simulink model "PPC_scheme_04072024_a"  (R2023b)
settings: Solver=FixedStepAuto  StartTime=0.0  StopTime=10.0  FixedStep=0.00025  RelTol=1e-3
libraries: slpidlib x1
settings Model: Creator=borgn  LastModifiedBy=borgn
settings SolverCC: ConcurrentTasks=on  PositivePriorityOrder=on
settings OptimizationCC: BlockReduction=off  OptimizeBlockIOStorage=off
settings DebuggingCC: TasksWithSamePriorityMsg=none
settings HardwareCC: ProdBitPerLong=64  ProdLongLongMode=on  ProdHWDeviceType=Intel->x86-64 (Linux 64)
settings RTWCC: Description=Simulink Real-Time  SystemTargetFile=slrealtime.tlc  TemplateMakefile=slrealtime_default_tmf  Toolchain=Simulink Real-Time Toolchain  BuildConfiguration=Faster Runs  CodeExecutionProfiling=on  TargetLang=C++

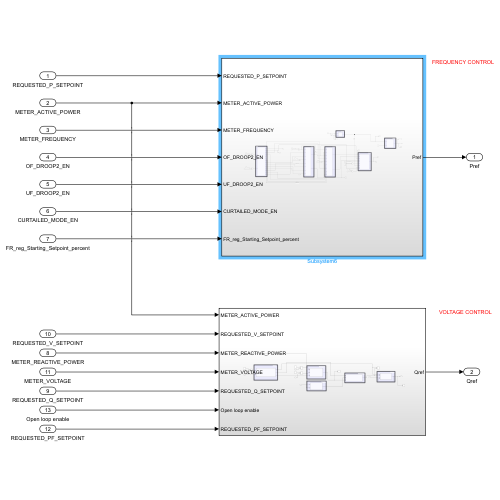
[thumbnail: Simulink's stored preview of the top-level diagram]
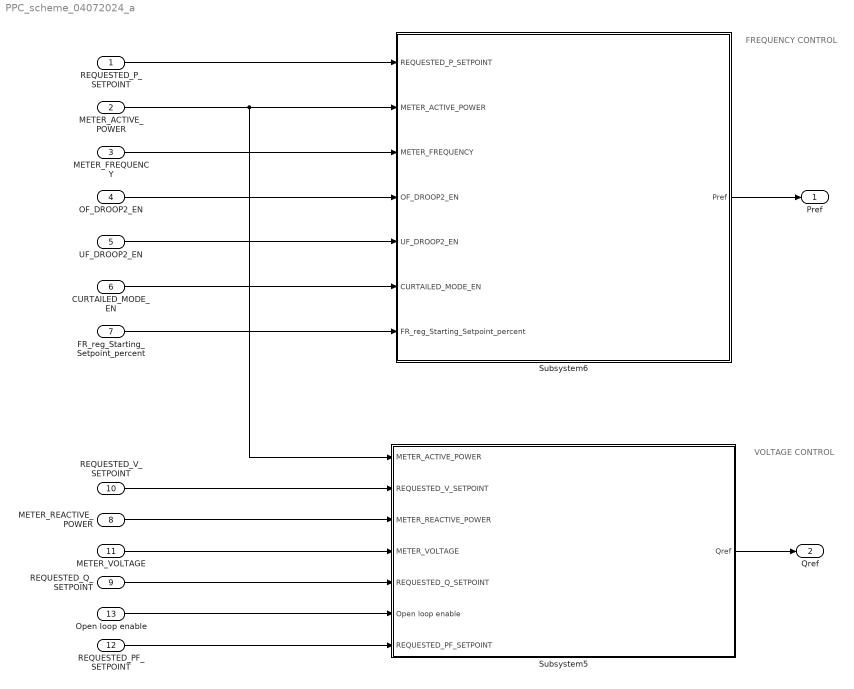
== system PPC_scheme_04072024_a ==
  note: FREQUENCY CONTROL
  note: VOLTAGE CONTROL
  REQUESTED_P_SETPOINT : Inport
  METER_ACTIVE_POWER : Inport  Port=2
  METER_FREQUENCY : Inport  Port=3
  OF_DROOP2_EN : Inport  Port=4
  UF_DROOP2_EN : Inport  Port=5
  CURTAILED_MODE_EN : Inport  Port=6
  FR_reg_Starting_Setpoint_percent : Inport  Port=7
  METER_REACTIVE_POWER : Inport  Port=8
  REQUESTED_Q_SETPOINT : Inport  Port=9
  REQUESTED_V_SETPOINT : Inport  Port=10
  METER_VOLTAGE : Inport  Port=11
  REQUESTED_PF_SETPOINT : Inport  Port=12
  Open loop enable : Inport  Port=13
  Subsystem5 : Subsystem
  Subsystem6 : Subsystem
  Pref : Outport
  Qref : Outport  Port=2
  wires:
  REQUESTED_P_SETPOINT/1 -> Subsystem6/1(REQUESTED_P_SETPOINT)
  METER_ACTIVE_POWER/1 -> Subsystem5/1(METER_ACTIVE_POWER), Subsystem6/2(METER_ACTIVE_POWER)
  METER_FREQUENCY/1 -> Subsystem6/3(METER_FREQUENCY)
  OF_DROOP2_EN/1 -> Subsystem6/4(OF_DROOP2_EN)
  UF_DROOP2_EN/1 -> Subsystem6/5(UF_DROOP2_EN)
  CURTAILED_MODE_EN/1 -> Subsystem6/6(CURTAILED_MODE_EN)
  FR_reg_Starting_Setpoint_percent/1 -> Subsystem6/7(FR_reg_Starting_Setpoint_percent)
  REQUESTED_V_SETPOINT/1 -> Subsystem5/2(REQUESTED_V_SETPOINT)
  METER_REACTIVE_POWER/1 -> Subsystem5/3(METER_REACTIVE_POWER)
  METER_VOLTAGE/1 -> Subsystem5/4(METER_VOLTAGE)
  REQUESTED_Q_SETPOINT/1 -> Subsystem5/5(REQUESTED_Q_SETPOINT)
  Open loop enable/1 -> Subsystem5/6(Open loop enable)
  REQUESTED_PF_SETPOINT/1 -> Subsystem5/7(REQUESTED_PF_SETPOINT)
  Subsystem6/1(Pref) -> Pref/1
  Subsystem5/1(Qref) -> Qref/1

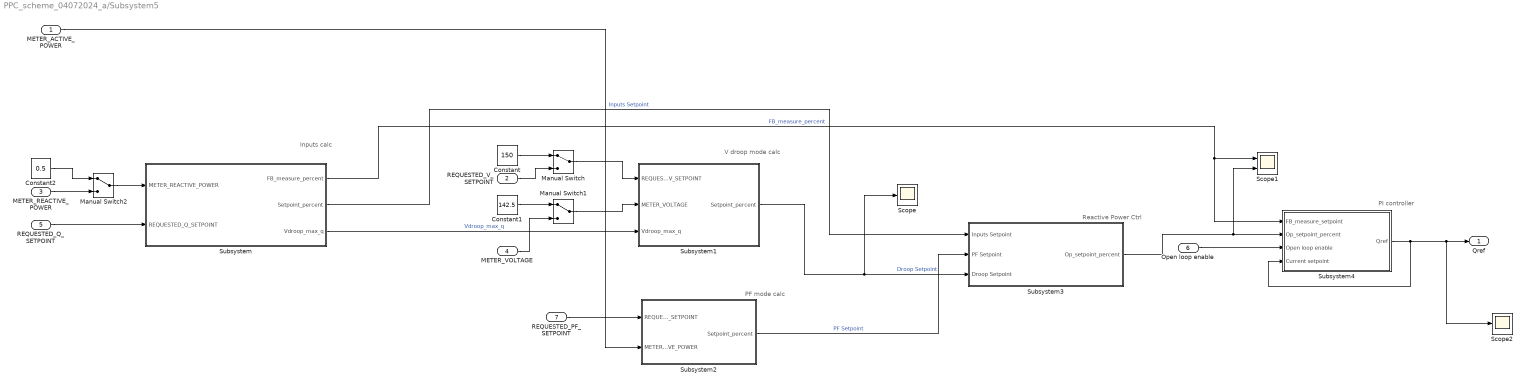
== system PPC_scheme_04072024_a/Subsystem5 ==
  note: PI controller
  note: Reactive Power Ctrl
  note: PF mode calc
  note: V droop mode calc
  note: Inputs calc
  METER_ACTIVE_POWER : Inport
  REQUESTED_V_SETPOINT : Inport  Port=2
  METER_REACTIVE_POWER : Inport  Port=3
  METER_VOLTAGE : Inport  Port=4
  REQUESTED_Q_SETPOINT : Inport  Port=5
  Open loop enable : Inport  Port=6
  REQUESTED_PF_SETPOINT : Inport  Port=7
  Constant : Constant  Value=150
  Constant1 : Constant  Value=142.5
  Constant2 : Constant  Value=0.5
  Manual Switch : ManualSwitch
  Manual Switch1 : ManualSwitch
  Manual Switch2 : ManualSwitch
  Scope : Scope
  Scope1 : Scope  NumInputPorts=2
  Scope2 : Scope
  Subsystem : Subsystem
  Subsystem1 : Subsystem
  Subsystem2 : Subsystem
  Subsystem3 : Subsystem
  Subsystem4 : Subsystem
  Qref : Outport
  wires:
  Subsystem/1(FB_measure_percent) -> Subsystem4/1(FB_measure_setpoint), Scope1/1  "FB_measure_percent"
  Subsystem4/1(Qref) -> Scope2/1, Qref/1, Subsystem4/4(Current setpoint)
  Subsystem/2(Setpoint_percent) -> Subsystem3/1(Inputs Setpoint)  "Inputs Setpoint"
  Subsystem1/1(Setpoint_percent) -> Scope/1, Subsystem3/3(Droop Setpoint)  "Droop Setpoint"
  REQUESTED_Q_SETPOINT/1 -> Subsystem/2(REQUESTED_Q_SETPOINT)
  Subsystem/3(Vdroop_max_q) -> Subsystem1/3(Vdroop_max_q)  "Vdroop_max_q"
  REQUESTED_PF_SETPOINT/1 -> Subsystem2/1(REQUESTED_PF_SETPOINT)
  Subsystem2/1(Setpoint_percent) -> Subsystem3/2(PF Setpoint)  "PF Setpoint"
  Subsystem3/1(Op_setpoint_percent) -> Scope1/2, Subsystem4/2(Op_setpoint_percent)
  Open loop enable/1 -> Subsystem4/3(Open loop enable)
  METER_ACTIVE_POWER/1 -> Subsystem2/2(METER_ACTIVE_POWER)
  REQUESTED_V_SETPOINT/1 -> Manual Switch/2
  Manual Switch/1 -> Subsystem1/1(REQUESTED_V_SETPOINT)
  Constant/1 -> Manual Switch/1
  Manual Switch1/1 -> Subsystem1/2(METER_VOLTAGE)
  METER_VOLTAGE/1 -> Manual Switch1/2
  Constant1/1 -> Manual Switch1/1
  METER_REACTIVE_POWER/1 -> Manual Switch2/2
  Manual Switch2/1 -> Subsystem/1(METER_REACTIVE_POWER)
  Constant2/1 -> Manual Switch2/1

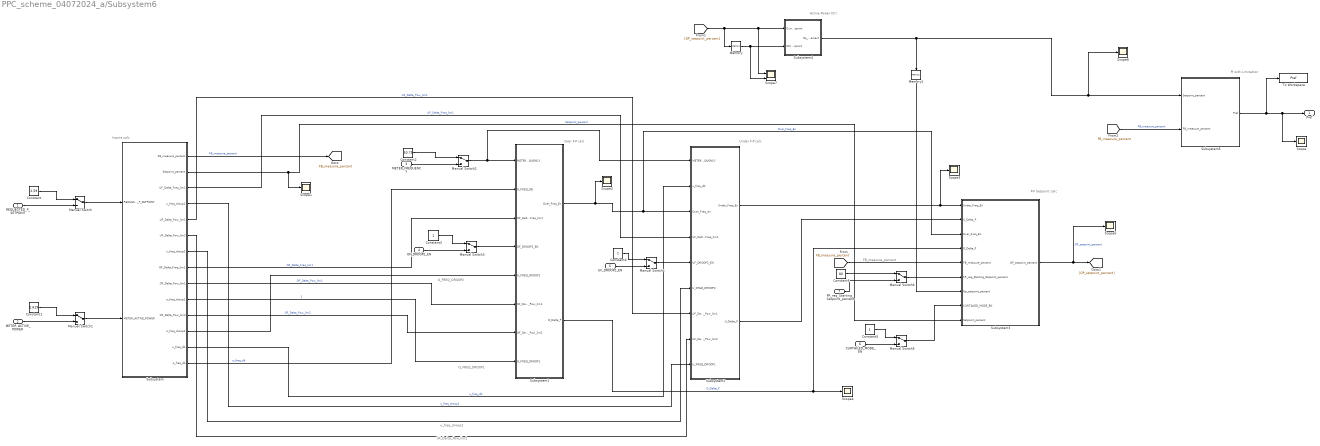
== system PPC_scheme_04072024_a/Subsystem6 ==
  note: PI with Limitation
  note: Active Power Ctrl
  note: FB_measure_percent
  note: P-F Setpoint calc
  note: UF_Delta_Pow_lim2
  note: u_freq_droop2
  note: Under F-P calc
  note: Inputs calc
  note: Over F-P calc
  note: O_FREQ_DROOP2
  note: O_FREQ_DROOP1
  REQUESTED_P_SETPOINT : Inport
  METER_ACTIVE_POWER : Inport  Port=2
  METER_FREQUENCY : Inport  Port=3
  OF_DROOP2_EN : Inport  Port=4
  UF_DROOP2_EN : Inport  Port=5
  CURTAILED_MODE_EN : Inport  Port=6
  FR_reg_Starting_Setpoint_percent : Inport  Port=7
  Constant : Constant  Value=2.59
  Constant1 : Constant  Value=1.619
  Constant2 : Constant  Value=50.75
  Constant3 : Constant
  Constant4 : Constant
  Constant5 : Constant
  Constant6 : Constant  Value=80
  Manual Switch{,1..6} (7 alike) : ManualSwitch
  Memory : Memory
  Memory1 : Memory
  Scope{,1..6} (7 alike) : Scope
  Scope7 : Scope  NumInputPorts=2
  Subsystem : Subsystem
  Subsystem1 : Subsystem
  Subsystem2 : Subsystem
  Subsystem3 : Subsystem
  Subsystem4 : Subsystem
  Subsystem5 : Subsystem
  To Workspace : ToWorkspace  VariableName=Pref  SaveFormat=Timeseries  SampleTime=-1
  Pref : Outport
  tag scope: FB_measure_percent=global
  wires:
  Constant1/1 -> Manual Switch1/1
  Manual Switch5/1 -> Subsystem3/8(CURTAILED_MODE_EN)
  Manual Switch6/1 -> Subsystem3/6(FR_reg_Starting_Setpoint_percent)
  Subsystem/11(OF_Delta_Pow_lim2) -> Subsystem1/7(OF_Delta_Pow_lim2)  "OF_Delta_Pow_lim2"
  CURTAILED_MODE_EN/1 -> Manual Switch5/2
  Manual Switch/1 -> Subsystem/1(REQUESTED_P_SETPOINT)
  Subsystem/9(OF_Delta_Pow_lim1) -> Subsystem1/6(OF_Delta_Pow_lim1)  "OF_Delta_Pow_lim1"
  Subsystem4/1(Op_setpoint_percent) -> Memory1/1, Scope6/1, Subsystem5/1(Setpoint_percent)
  Subsystem/1(FB_measure_percent) -> [FB_measure_percent]  "FB_measure_percent"
  Subsystem/14(o_freq_db) -> Subsystem1/2(O_FREQ_DB)  "o_freq_db"
  Subsystem/5(UF_Delta_Pow_lim1) -> Subsystem2/7(UF_Delta_Pow_lim1)  "UF_Delta_Pow_lim1"
  Subsystem2/1(Under_Freq_En) -> Scope3/1, Subsystem3/1(Under_Freq_En)
  Manual Switch1/1 -> Subsystem/2(METER_ACTIVE_POWER)
  [OP_setpoint_percent] -> Memory/1, Scope7/1, Subsystem4/1(Current Setpoint)
  OF_DROOP2_EN/1 -> Manual Switch3/2
  Subsystem/13(u_freq_db) -> Subsystem2/2(u_freq_db)  "u_freq_db"
  Memory1/1 -> Subsystem3/7(Op_setpoint_percent)
  Subsystem/12(o_freq_droop2) -> Subsystem1/5(O_FREQ_DROOP2)
  Subsystem/8(OF_Delta_Freq_lim1) -> Subsystem1/3(OF_Delta_Freq_lim1)  "OF_Delta_Freq_lim1"
  Constant5/1 -> Manual Switch5/1
  Subsystem5/1(Pref) -> To Workspace/1, Pref/1, Scope/1
  Constant/1 -> Manual Switch/1
  Manual Switch2/1 -> Subsystem2/1(METER_FREQUENCY), Subsystem1/1(METER_FREQUENCY)
  FR_reg_Starting_Setpoint_percent/1 -> Manual Switch6/2
  Subsystem/4(u_freq_droop1) -> Subsystem2/9(U_FREQ_DROOP1)  "u_freq_droop1"
  METER_ACTIVE_POWER/1 -> Manual Switch1/2
  UF_DROOP2_EN/1 -> Manual Switch4/2
  Subsystem/3(UF_Delta_Freq_lim1) -> Subsystem2/4(UF_Delta_Freq_lim1)  "UF_Delta_Freq_lim1"
  Subsystem/10(o_freq_droop1) -> Subsystem1/8(O_FREQ_DROOP1)  "1"
  REQUESTED_P_SETPOINT/1 -> Manual Switch/2
  Subsystem1/1(Over_Freq_En) -> Scope2/1, Subsystem3/3(Over_Freq_En), Subsystem2/3(Over_Freq_en)  "Over_Freq_En"
  [FB_measure_percent] -> Subsystem3/5(FB_measure_percent)
  [FB_measure_percent] -> Subsystem5/2(FB_measure_percent)  "FB_measure_percent"
  Manual Switch4/1 -> Subsystem2/5(UF_DROOP2_EN)
  METER_FREQUENCY/1 -> Manual Switch2/2
  Subsystem1/2(O_Delta_P) -> Subsystem3/4(O_Delta_P), Scope4/1  "O_Delta_P"
  Constant3/1 -> Manual Switch3/1
  Subsystem2/2(U_Delta_P) -> Subsystem3/2(U_Delta_P)
  Memory/1 -> Scope7/2, Subsystem4/2(Old Setpoint)
  Subsystem/6(UF_Delta_Pow_lim2) -> Subsystem2/8(UF_Delta_Pow_lim2)
  Constant2/1 -> Manual Switch2/1
  Constant4/1 -> Manual Switch4/1
  Subsystem/2(Setpoint_percent) -> Scope1/1, Subsystem3/9(Setpoint_percent)  "Setpoint_percent"
  Subsystem/7(u_freq_droop2) -> Subsystem2/6(U_FREQ_DROOP2)
  Manual Switch3/1 -> Subsystem1/4(OF_DROOP2_EN)
  Subsystem3/1(OP_setpoint_percent) -> Scope5/1, [OP_setpoint_percent]  "OP_setpoint_percent"
  Constant6/1 -> Manual Switch6/1

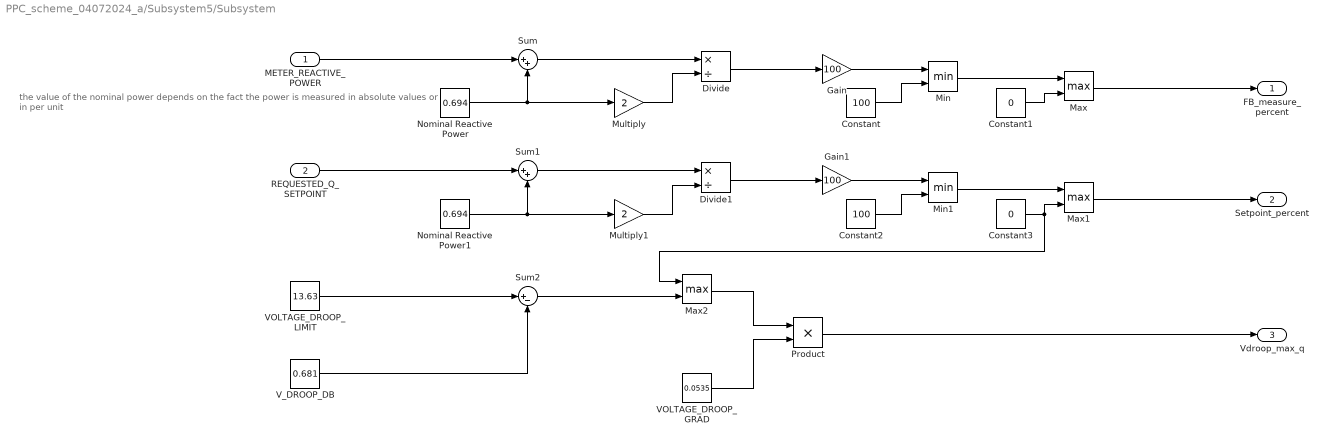
== system PPC_scheme_04072024_a/Subsystem5/Subsystem ==
  note: the value of the nominal power depends on the fact the power is measured in absolute values or in per unit
  METER_REACTIVE_POWER : Inport
  REQUESTED_Q_SETPOINT : Inport  Port=2
  Constant : Constant  Value=100
  Constant1 : Constant  Value=0
  Constant2 : Constant  Value=100
  Constant3 : Constant  Value=0
  Divide : Product  Inputs=*/
  Divide1 : Product  Inputs=*/
  Gain : Gain  Gain=100
  Gain1 : Gain  Gain=100
  Max : MinMax  Function=max  Inputs=2
  Max1 : MinMax  Function=max  Inputs=2
  Max2 : MinMax  Function=max  Inputs=2
  Min : MinMax  Inputs=2
  Min1 : MinMax  Inputs=2
  Multiply : Gain  Gain=2
  Multiply1 : Gain  Gain=2
  Nominal Reactive Power : Constant  Value=0.694
  Nominal Reactive Power1 : Constant  Value=0.694
  Product : Product
  Sum : Sum  Inputs=|++
  Sum1 : Sum  Inputs=|++
  Sum2 : Sum  Inputs=|+-
  VOLTAGE_DROOP_GRAD : Constant  Value=0.0535
  VOLTAGE_DROOP_LIMIT : Constant  Value=13.63
  V_DROOP_DB : Constant  Value=0.681
  FB_measure_percent : Outport
  Setpoint_percent : Outport  Port=2
  Vdroop_max_q : Outport  Port=3
  wires:
  Gain/1 -> Min/1
  Constant1/1 -> Max/2
  Max/1 -> FB_measure_percent/1
  Nominal Reactive Power/1 -> Multiply/1, Sum/2
  METER_REACTIVE_POWER/1 -> Sum/1
  Multiply/1 -> Divide/2
  Min/1 -> Max/1
  Sum/1 -> Divide/1
  Constant/1 -> Min/2
  Divide/1 -> Gain/1
  Multiply1/1 -> Divide1/2
  Constant2/1 -> Min1/2
  Sum1/1 -> Divide1/1
  REQUESTED_Q_SETPOINT/1 -> Sum1/1
  Nominal Reactive Power1/1 -> Multiply1/1, Sum1/2
  Min1/1 -> Max1/1
  Constant3/1 -> Max2/1, Max1/2
  Divide1/1 -> Gain1/1
  Gain1/1 -> Min1/1
  Max1/1 -> Setpoint_percent/1
  VOLTAGE_DROOP_LIMIT/1 -> Sum2/1
  V_DROOP_DB/1 -> Sum2/2
  Sum2/1 -> Max2/2
  Max2/1 -> Product/1
  VOLTAGE_DROOP_GRAD/1 -> Product/2
  Product/1 -> Vdroop_max_q/1

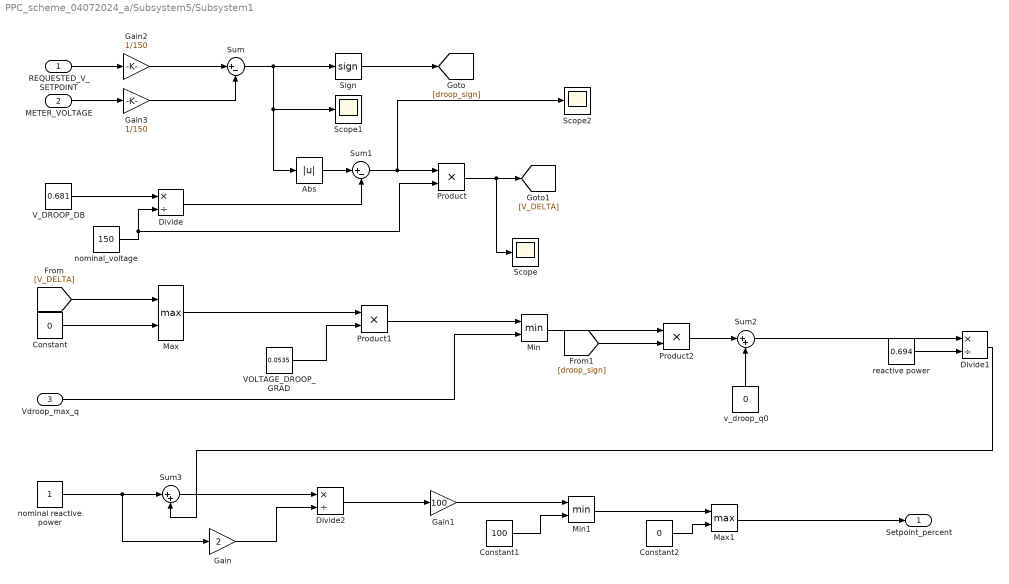
== system PPC_scheme_04072024_a/Subsystem5/Subsystem1 ==
  REQUESTED_V_SETPOINT : Inport
  METER_VOLTAGE : Inport  Port=2
  Vdroop_max_q : Inport  Port=3
  " reactive power" : Constant  Value=0.694
  Abs : Abs  SaturateOnIntegerOverflow=off
  Constant : Constant  Value=0
  Constant1 : Constant  Value=100
  Constant2 : Constant  Value=0
  Divide : Product  Inputs=*/
  Divide1 : Product  Inputs=*/
  Divide2 : Product  Inputs=*/
  Gain : Gain  Gain=2
  Gain1 : Gain  Gain=100
  Gain2 : Gain  Gain=1/150
  Gain3 : Gain  Gain=1/150
  Max : MinMax  Function=max  Inputs=2
  Max1 : MinMax  Function=max  Inputs=2
  Min : MinMax  Inputs=2
  Min1 : MinMax  Inputs=2
  Product : Product
  Product1 : Product
  Product2 : Product
  Scope : Scope
  Scope1 : Scope
  Scope2 : Scope
  Sign : Signum
  Sum : Sum  Inputs=|+-
  Sum1 : Sum  Inputs=|+-
  Sum2 : Sum  Inputs=|++
  Sum3 : Sum  Inputs=|++
  VOLTAGE_DROOP_GRAD : Constant  Value=0.0535
  V_DROOP_DB : Constant  Value=0.681
  nominal reactive power : Constant
  nominal_voltage : Constant  Value=150
  v_droop_q0 : Constant  Value=0
  Setpoint_percent : Outport
  wires:
  V_DROOP_DB/1 -> Divide/1
  Constant/1 -> Max/2
  Divide/1 -> Sum1/2
  Sum1/1 -> Scope2/1, Product/1
  nominal_voltage/1 -> Product/2, Divide/2
  Abs/1 -> Sum1/1
  Product/1 -> Scope/1, [V_DELTA]
  [V_DELTA] -> Max/1
  Sign/1 -> [droop_sign]
  Max/1 -> Product1/1
  VOLTAGE_DROOP_GRAD/1 -> Product1/2
  Product1/1 -> Min/1
  Vdroop_max_q/1 -> Min/2
  Min/1 -> Product2/1
  [droop_sign] -> Product2/2
  Product2/1 -> Sum2/1
  v_droop_q0/1 -> Sum2/2
  Sum2/1 -> Divide1/1
  " reactive power"/1 -> Divide1/2
  Divide1/1 -> Sum3/2
  nominal reactive power/1 -> Gain/1, Sum3/1
  Sum3/1 -> Divide2/1
  Gain/1 -> Divide2/2
  Divide2/1 -> Gain1/1
  Gain1/1 -> Min1/1
  Constant1/1 -> Min1/2
  Min1/1 -> Max1/1
  Constant2/1 -> Max1/2
  Max1/1 -> Setpoint_percent/1
  REQUESTED_V_SETPOINT/1 -> Gain2/1
  METER_VOLTAGE/1 -> Gain3/1
  Gain2/1 -> Sum/1
  Gain3/1 -> Sum/2
  Sum/1 -> Abs/1, Scope1/1, Sign/1

== system PPC_scheme_04072024_a/Subsystem5/Subsystem2 ==
  REQUESTED_PF_SETPOINT : Inport
  METER_ACTIVE_POWER : Inport  Port=2
  Constant : Constant  Value=100
  Constant1 : Constant  Value=0
  Divide : Product  Inputs=*/
  Divide1 : Product  Inputs=*/
  Gain : Gain  Gain=2
  Gain1 : Gain  Gain=100
  Max : MinMax  Function=max  Inputs=2
  Min : MinMax  Inputs=2
  Product : Product
  Sin : Trigonometry  Operator=acos
  Sum : Sum  Inputs=|++
  Tan : Trigonometry  Operator=tan
  nominal active power : Constant  Value=3.238
  nominal reactive power : Constant
  Setpoint_percent : Outport
  wires:
  REQUESTED_PF_SETPOINT/1 -> Sin/1
  METER_ACTIVE_POWER/1 -> Divide/1
  Sin/1 -> Tan/1
  nominal active power/1 -> Divide/2
  Tan/1 -> Product/1
  Divide/1 -> Product/2
  Product/1 -> Sum/1
  nominal reactive power/1 -> Gain/1, Sum/2
  Sum/1 -> Divide1/1
  Gain/1 -> Divide1/2
  Divide1/1 -> Gain1/1
  Gain1/1 -> Min/2
  Constant/1 -> Min/1
  Min/1 -> Max/1
  Constant1/1 -> Max/2
  Max/1 -> Setpoint_percent/1

== system PPC_scheme_04072024_a/Subsystem5/Subsystem3 ==
  Inputs Setpoint : Inport
  PF Setpoint : Inport  Port=2
  Droop Setpoint : Inport  Port=3
  MATLAB Function : MATLAB Function  TreatAsAtomicUnit=on
  Mux : Mux
  control mode : Constant  Value=3
  Op_setpoint_percent : Outport
  wires:
  MATLAB Function/1(y) -> Op_setpoint_percent/1
  Inputs Setpoint/1 -> Mux/2
  Mux/1 -> MATLAB Function/1(u)
  PF Setpoint/1 -> Mux/3
  Droop Setpoint/1 -> Mux/4
  control mode/1 -> Mux/1

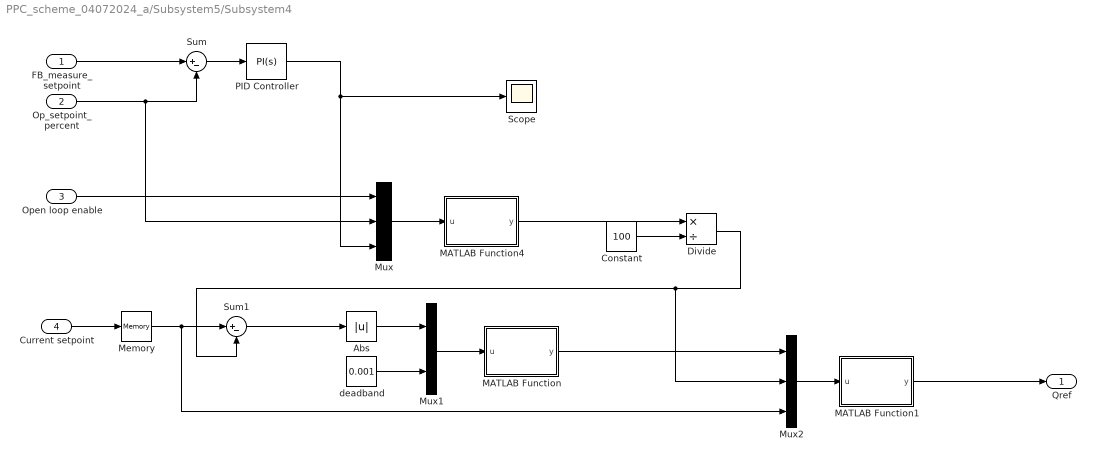
== system PPC_scheme_04072024_a/Subsystem5/Subsystem4 ==
  FB_measure_setpoint : Inport
  Op_setpoint_percent : Inport  Port=2
  Open loop enable : Inport  Port=3
  Current setpoint : Inport  Port=4
  Abs : Abs  SaturateOnIntegerOverflow=off
  Constant : Constant  Value=100
  Divide : Product  Inputs=*/
  MATLAB Function : MATLAB Function  TreatAsAtomicUnit=on
  MATLAB Function1 : MATLAB Function  TreatAsAtomicUnit=on
  MATLAB Function4 : MATLAB Function  TreatAsAtomicUnit=on
  Memory : Memory
  Mux : Mux  Inputs=3
  Mux1 : Mux  Inputs=2
  Mux2 : Mux  Inputs=3
  PID Controller : slpidlib/PID Controller  Controller=PI  Form=Parallel  TimeDomain=Continuous-time  UseExternalTs=off  SampleTime=-1  IntegratorMethod=Forward Euler  FilterMethod=Forward Euler  ControllerParametersSource=internal  P=1  I=0.05  UseKiTs=off  D=0  N=100  UseFilter=on  TunerSelectOption=Transfer Function Based (PID Tuner App)  InitialConditionSource=internal  InitialConditionForIntegrator=0  InitialConditionForFilter=0  DifferentiatorICPrevScaledInput=0  ExternalReset=none  TrackingMode=off  Kt=1  LimitOutput=on  SatLimitsSource=internal  UpperSaturationLimit=100  LowerSaturationLimit=-100  LinearizeAsGain=on  AntiWindupMode=none  Kb=1  LimitIntegrator=off  UpperIntegratorSaturationLimit=inf  LowerIntegratorSaturationLimit=-inf  POutMin=[]  POutMax=[]  IOutMin=[]  IOutMax=[]  DOutMin=[]  DOutMax=[]  NOutMin=[]  NOutMax=[]  SumOutMin=[]  SumOutMax=[]  SaturationOutMin=[]  SaturationOutMax=[]  PParamMin=[]  PParamMax=[]  IParamMin=[]  IParamMax=[]  DParamMin=[]  DParamMax=[]  NParamMin=[]  NParamMax=[]  KbParamMin=[]  KbParamMax=[]  KtParamMin=[]  KtParamMax=[]  KbOutMin=[]  KbOutMax=[]  KtOutMin=[]  KtOutMax=[]  IntegratorOutMin=[]  IntegratorOutMax=[]  FilterOutMin=[]  FilterOutMax=[]  SumI1OutMin=[]  SumI1OutMax=[]  SumI2OutMin=[]  SumI2OutMax=[]  SumI3OutMin=[]  SumI3OutMax=[]  SumI4OutMin=[]  SumI4OutMax=[]  SumDOutMin=[]  SumDOutMax=[]  DifferentiatorOutMin=[]  DifferentiatorOutMax=[]  FilterDiffOutCoefMin=[]  FilterDiffOutCoefMax=[]  ReciprocalOutMin=[]  ReciprocalOutMax=[]  SumDenOutMin=[]  SumDenOutMax=[]  SumNumOutMin=[]  SumNumOutMax=[]  DivideOutMin=[]  DivideOutMax=[]  UdiffTsProdOutMin=[]  UdiffTsProdOutMax=[]  NTsProdOutMin=[]  NTsProdOutMax=[]  UintegralTsProdOutMin=[]  UintegralTsProdOutMax=[]  UngainTsProdOutMin=[]  UngainTsProdOutMax=[]  ClampingZeroOutDataTypeStr=Inherit: Inherit via back propagation  ClampingZeroOutMin=[]  ClampingZeroOutMax=[]  FilterDenConstantOutDataTypeStr=Inherit: Inherit via back propagation  FilterDenConstantOutMin=[]  FilterDenConstantOutMax=[]  PCopyOutDataTypeStr=Inherit: Inherit via back propagation  PCopyOutMin=[]  PCopyOutMax=[]  NCopyOutDataTypeStr=Inherit: Inherit via back propagation  NCopyOutMin=[]  NCopyOutMax=[]  IntegratorContinuousStateAttributes=''  IntegratorStateMustResolveToSignalObject=off  IntegratorRTWStateStorageClass=Auto  FilterContinuousStateAttributes=''  FilterStateMustResolveToSignalObject=off  FilterRTWStateStorageClass=Auto  ParallelPVariant=InternalParameters  IdealPVariant=Disabled  IVariant=InternalParameters  DVariant=Disabled  IntegratorVariant=Continuous  SatVariant=Enabled  AWVariant=Passthrough  PCopyVariant=Disabled  TRVariant=Disabled  FdbkBlocksVariant=Forward  IdealPFdbkVariant=Disabled  SatFdbkVariant=Disabled  DerivativeFilterVariant=Disabled  NVariant=Disabled  NCopyVariant=Disabled_SignalSpec  FilterICVariant=Disabled  IntegratorICVariant=InternalICs  ExternalResetVariant=Disabled  TRSumVariant=Passthrough  SumFdbkVariant=Disabled  SumVariant=Sum_PI  TsampFilterVariant=InternalTs  TsampNgainVariant=Passthrough  TsampIntegralVariant=Disabled_SignalSpec  ExternalSaturationOutDataTypeStr=Inherit: Same as second input
  Scope : Scope
  Sum : Sum  Inputs=|+-
  Sum1 : Sum  Inputs=|+-
  deadband : Constant  Value=0.001
  Qref : Outport
  wires:
  Op_setpoint_percent/1 -> Mux/2, Sum/2
  Sum/1 -> PID Controller/1
  FB_measure_setpoint/1 -> Sum/1
  PID Controller/1 -> Scope/1, Mux/3
  Open loop enable/1 -> Mux/1
  Mux/1 -> MATLAB Function4/1(u)
  MATLAB Function4/1(y) -> Divide/1
  Constant/1 -> Divide/2
  Divide/1 -> Mux2/2, Sum1/2
  Sum1/1 -> Abs/1
  Abs/1 -> Mux1/1
  deadband/1 -> Mux1/2
  Mux1/1 -> MATLAB Function/1(u)
  MATLAB Function/1(y) -> Mux2/1
  Mux2/1 -> MATLAB Function1/1(u)
  MATLAB Function1/1(y) -> Qref/1
  Current setpoint/1 -> Memory/1
  Memory/1 -> Mux2/3, Sum1/1

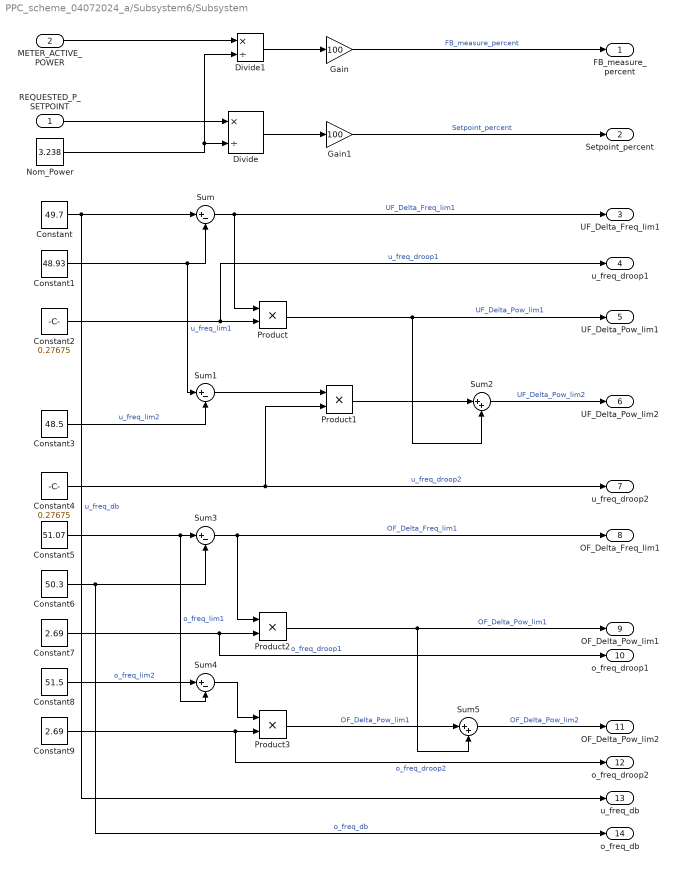
== system PPC_scheme_04072024_a/Subsystem6/Subsystem ==
  REQUESTED_P_SETPOINT : Inport
  METER_ACTIVE_POWER : Inport  Port=2
  Constant : Constant  Value=49.7
  Constant1 : Constant  Value=48.93
  Constant2 : Constant  Value=0.27675
  Constant3 : Constant  Value=48.5
  Constant4 : Constant  Value=0.27675
  Constant5 : Constant  Value=51.07
  Constant6 : Constant  Value=50.3
  Constant7 : Constant  Value=2.69
  Constant8 : Constant  Value=51.5
  Constant9 : Constant  Value=2.69
  Divide : Product  Inputs=*/
  Divide1 : Product  Inputs=*/
  Gain : Gain  Gain=100
  Gain1 : Gain  Gain=100
  Nom_Power : Constant  Value=3.238
  Product{,1..3} (4 alike) : Product
  Sum{,1,3..4} (4 alike) : Sum  Inputs=|+-
  Sum2 : Sum  Inputs=|++
  Sum5 : Sum  Inputs=|++
  FB_measure_percent : Outport
  Setpoint_percent : Outport  Port=2
  UF_Delta_Freq_lim1 : Outport  Port=3
  u_freq_droop1 : Outport  Port=4
  UF_Delta_Pow_lim1 : Outport  Port=5
  UF_Delta_Pow_lim2 : Outport  Port=6
  u_freq_droop2 : Outport  Port=7
  OF_Delta_Freq_lim1 : Outport  Port=8
  OF_Delta_Pow_lim1 : Outport  Port=9
  o_freq_droop1 : Outport  Port=10
  OF_Delta_Pow_lim2 : Outport  Port=11
  o_freq_droop2 : Outport  Port=12
  u_freq_db : Outport  Port=13
  o_freq_db : Outport  Port=14
  wires:
  Gain/1 -> FB_measure_percent/1  "FB_measure_percent"
  Constant5/1 -> Sum4/2, Sum3/1  "o_freq_lim1"
  Sum/1 -> UF_Delta_Freq_lim1/1, Product/1  "UF_Delta_Freq_lim1"
  REQUESTED_P_SETPOINT/1 -> Divide/1
  Constant7/1 -> o_freq_droop1/1, Product2/2  "o_freq_droop1"
  Product/1 -> UF_Delta_Pow_lim1/1, Sum2/2  "UF_Delta_Pow_lim1"
  Sum5/1 -> OF_Delta_Pow_lim2/1  "OF_Delta_Pow_lim2"
  Nom_Power/1 -> Divide1/2, Divide/2
  Product2/1 -> OF_Delta_Pow_lim1/1, Sum5/2  "OF_Delta_Pow_lim1"
  Constant9/1 -> o_freq_droop2/1, Product3/2  "o_freq_droop2"
  Product1/1 -> Sum2/1
  Sum2/1 -> UF_Delta_Pow_lim2/1  "UF_Delta_Pow_lim2"
  Constant4/1 -> u_freq_droop2/1, Product1/2  "u_freq_droop2"
  Sum4/1 -> Product3/1
  Constant2/1 -> u_freq_droop1/1, Product/2  "u_freq_droop1"
  Constant1/1 -> Sum1/1, Sum/2  "u_freq_lim1"
  Product3/1 -> Sum5/1  "OF_Delta_Pow_lim1"
  Constant6/1 -> o_freq_db/1, Sum3/2  "o_freq_db"
  METER_ACTIVE_POWER/1 -> Divide1/1
  Constant/1 -> u_freq_db/1, Sum/1  "u_freq_db"
  Gain1/1 -> Setpoint_percent/1  "Setpoint_percent"
  Divide/1 -> Gain1/1
  Divide1/1 -> Gain/1
  Sum1/1 -> Product1/1
  Constant3/1 -> Sum1/2  "u_freq_lim2"
  Sum3/1 -> OF_Delta_Freq_lim1/1, Product2/1  "OF_Delta_Freq_lim1"
  Constant8/1 -> Sum4/1  "o_freq_lim2"

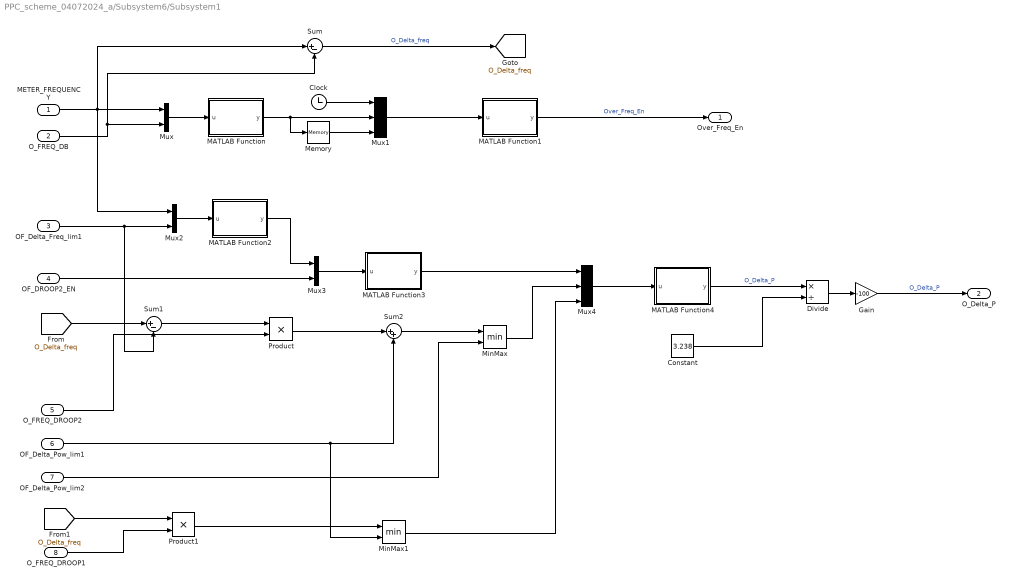
== system PPC_scheme_04072024_a/Subsystem6/Subsystem1 ==
  METER_FREQUENCY : Inport
  O_FREQ_DB : Inport  Port=2
  OF_Delta_Freq_lim1 : Inport  Port=3
  OF_DROOP2_EN : Inport  Port=4
  O_FREQ_DROOP2 : Inport  Port=5
  OF_Delta_Pow_lim1 : Inport  Port=6
  OF_Delta_Pow_lim2 : Inport  Port=7
  O_FREQ_DROOP1 : Inport  Port=8
  Clock : Clock
  Constant : Constant  Value=3.238
  Divide : Product  Inputs=*/
  Gain : Gain  Gain=-100
  MATLAB Function : MATLAB Function  TreatAsAtomicUnit=on
  MATLAB Function1 : MATLAB Function  TreatAsAtomicUnit=on
  MATLAB Function2 : MATLAB Function  TreatAsAtomicUnit=on
  MATLAB Function3 : MATLAB Function  TreatAsAtomicUnit=on
  MATLAB Function4 : MATLAB Function  TreatAsAtomicUnit=on
  Memory : Memory
  MinMax : MinMax  Inputs=2
  MinMax1 : MinMax  Inputs=2
  Mux : Mux  Inputs=2
  Mux1 : Mux  Inputs=3
  Mux2 : Mux  Inputs=2
  Mux3 : Mux  Inputs=2
  Mux4 : Mux  Inputs=3
  Product : Product
  Product1 : Product
  Sum : Sum  Inputs=|+-
  Sum1 : Sum  Inputs=|+-
  Sum2 : Sum  Inputs=|++
  Over_Freq_En : Outport
  O_Delta_P : Outport  Port=2
  tag scope: O_Delta_freq=global
  wires:
  Memory/1 -> Mux1/3
  Sum1/1 -> Product/1
  OF_Delta_Pow_lim2/1 -> MinMax/2
  OF_Delta_Pow_lim1/1 -> MinMax1/2, Sum2/2
  Sum/1 -> [O_Delta_freq]  "O_Delta_freq"
  Mux1/1 -> MATLAB Function1/1(u)
  MATLAB Function/1(y) -> Memory/1, Mux1/2
  Mux3/1 -> MATLAB Function3/1(u)
  MATLAB Function3/1(y) -> Mux4/1
  OF_Delta_Freq_lim1/1 -> Sum1/2, Mux2/2
  Clock/1 -> Mux1/1
  METER_FREQUENCY/1 -> Mux2/1, Sum/1, Mux/1
  Mux/1 -> MATLAB Function/1(u)
  MinMax1/1 -> Mux4/3
  O_FREQ_DROOP2/1 -> Product/2
  OF_DROOP2_EN/1 -> Mux3/2
  MATLAB Function2/1(y) -> Mux3/1
  O_FREQ_DROOP1/1 -> Product1/2
  O_FREQ_DB/1 -> Sum/2, Mux/2
  MATLAB Function1/1(y) -> Over_Freq_En/1  "Over_Freq_En"
  Mux2/1 -> MATLAB Function2/1(u)
  Mux4/1 -> MATLAB Function4/1(u)
  [O_Delta_freq] -> Sum1/1
  Sum2/1 -> MinMax/1
  Product1/1 -> MinMax1/1
  MinMax/1 -> Mux4/2
  Product/1 -> Sum2/1
  [O_Delta_freq] -> Product1/1
  MATLAB Function4/1(y) -> Divide/1  "O_Delta_P"
  Constant/1 -> Divide/2
  Divide/1 -> Gain/1
  Gain/1 -> O_Delta_P/1  "O_Delta_P"

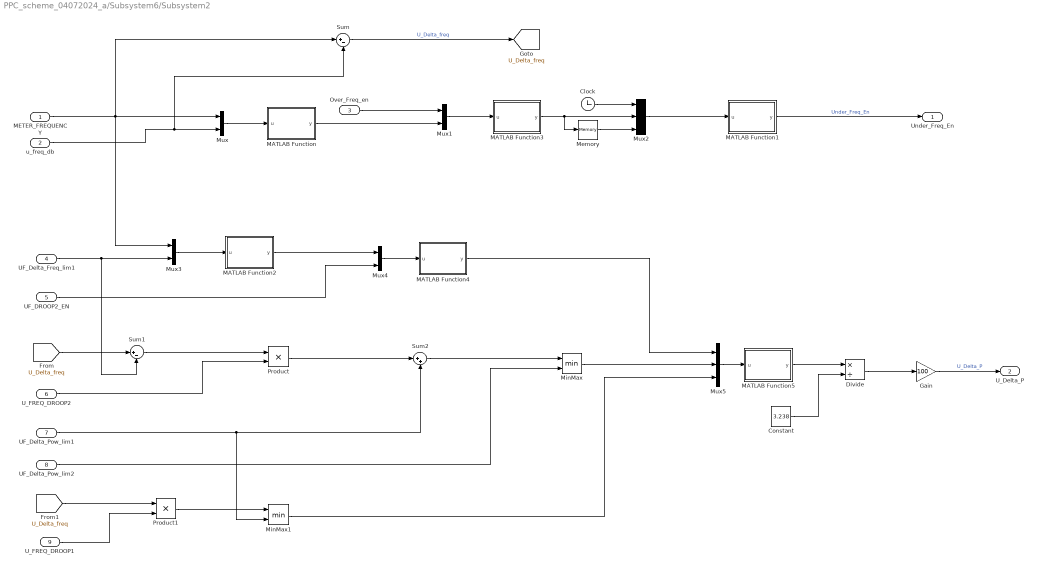
== system PPC_scheme_04072024_a/Subsystem6/Subsystem2 ==
  METER_FREQUENCY : Inport
  u_freq_db : Inport  Port=2
  Over_Freq_en : Inport  Port=3
  UF_Delta_Freq_lim1 : Inport  Port=4
  UF_DROOP2_EN : Inport  Port=5
  U_FREQ_DROOP2 : Inport  Port=6
  UF_Delta_Pow_lim1 : Inport  Port=7
  UF_Delta_Pow_lim2 : Inport  Port=8
  U_FREQ_DROOP1 : Inport  Port=9
  Clock : Clock
  Constant : Constant  Value=3.238
  Divide : Product  Inputs=*/
  Gain : Gain  Gain=100
  MATLAB Function : MATLAB Function  TreatAsAtomicUnit=on
  MATLAB Function1 : MATLAB Function  TreatAsAtomicUnit=on
  MATLAB Function2 : MATLAB Function  TreatAsAtomicUnit=on
  MATLAB Function3 : MATLAB Function  TreatAsAtomicUnit=on
  MATLAB Function4 : MATLAB Function  TreatAsAtomicUnit=on
  MATLAB Function5 : MATLAB Function  TreatAsAtomicUnit=on
  Memory : Memory
  MinMax : MinMax  Inputs=2
  MinMax1 : MinMax  Inputs=2
  Mux{,1,3..4} (4 alike) : Mux  Inputs=2
  Mux2 : Mux  Inputs=3
  Mux5 : Mux  Inputs=3
  Product : Product
  Product1 : Product
  Sum : Sum  Inputs=|+-
  Sum1 : Sum  Inputs=|+-
  Sum2 : Sum  Inputs=|++
  Under_Freq_En : Outport
  U_Delta_P : Outport  Port=2
  tag scope: U_Delta_freq=global
  wires:
  Mux/1 -> MATLAB Function/1(u)
  u_freq_db/1 -> Sum/2, Mux/2
  METER_FREQUENCY/1 -> Mux3/1, Sum/1, Mux/1
  MATLAB Function/1(y) -> Mux1/2
  Over_Freq_en/1 -> Mux1/1
  Mux1/1 -> MATLAB Function3/1(u)
  MATLAB Function1/1(y) -> Under_Freq_En/1  "Under_Freq_En"
  Clock/1 -> Mux2/1
  Memory/1 -> Mux2/3
  MATLAB Function3/1(y) -> Memory/1, Mux2/2
  Mux2/1 -> MATLAB Function1/1(u)
  Sum/1 -> [U_Delta_freq]  "U_Delta_freq"
  UF_Delta_Freq_lim1/1 -> Sum1/2, Mux3/2
  Mux3/1 -> MATLAB Function2/1(u)
  MATLAB Function2/1(y) -> Mux4/1
  UF_DROOP2_EN/1 -> Mux4/2
  Mux4/1 -> MATLAB Function4/1(u)
  [U_Delta_freq] -> Sum1/1
  Sum1/1 -> Product/1
  U_FREQ_DROOP2/1 -> Product/2
  Product/1 -> Sum2/1
  UF_Delta_Pow_lim1/1 -> MinMax1/2, Sum2/2
  Sum2/1 -> MinMax/1
  UF_Delta_Pow_lim2/1 -> MinMax/2
  [U_Delta_freq] -> Product1/1
  U_FREQ_DROOP1/1 -> Product1/2
  Product1/1 -> MinMax1/1
  MATLAB Function4/1(y) -> Mux5/1
  MinMax/1 -> Mux5/2
  MinMax1/1 -> Mux5/3
  Mux5/1 -> MATLAB Function5/1(u)
  MATLAB Function5/1(y) -> Divide/1
  Constant/1 -> Divide/2
  Divide/1 -> Gain/1
  Gain/1 -> U_Delta_P/1  "U_Delta_P"

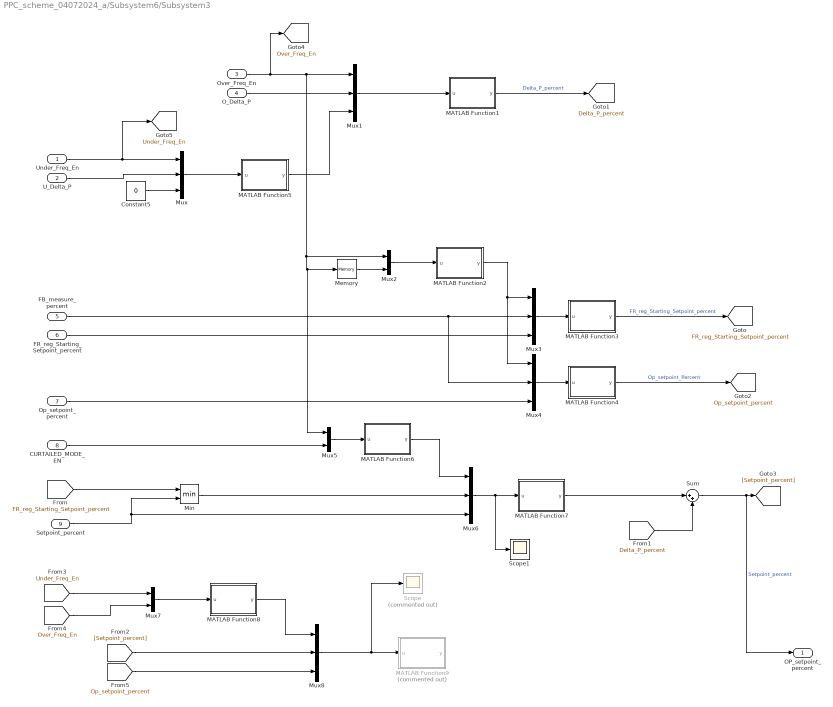
== system PPC_scheme_04072024_a/Subsystem6/Subsystem3 ==
  Under_Freq_En : Inport
  U_Delta_P : Inport  Port=2
  Over_Freq_En : Inport  Port=3
  O_Delta_P : Inport  Port=4
  FB_measure_percent : Inport  Port=5
  FR_reg_Starting_Setpoint_percent : Inport  Port=6
  Op_setpoint_percent : Inport  Port=7
  CURTAILED_MODE_EN : Inport  Port=8
  Setpoint_percent : Inport  Port=9
  Constant5 : Constant  Value=0
  MATLAB Function1 : MATLAB Function  TreatAsAtomicUnit=on
  MATLAB Function2 : MATLAB Function  TreatAsAtomicUnit=on
  MATLAB Function3 : MATLAB Function  TreatAsAtomicUnit=on
  MATLAB Function4 : MATLAB Function  TreatAsAtomicUnit=on
  MATLAB Function5 : MATLAB Function  TreatAsAtomicUnit=on
  MATLAB Function6 : MATLAB Function  TreatAsAtomicUnit=on
  MATLAB Function7 : MATLAB Function  TreatAsAtomicUnit=on
  MATLAB Function8 : MATLAB Function  TreatAsAtomicUnit=on
  MATLAB Function9 : MATLAB Function  Commented=on  TreatAsAtomicUnit=on
  Memory : Memory
  Min : MinMax  Inputs=2
  Mux{,1,3..4,6,8} (6 alike) : Mux  Inputs=3
  Mux2 : Mux  Inputs=2
  Mux5 : Mux  Inputs=2
  Mux7 : Mux  Inputs=2
  Scope : Scope  Commented=on
  Scope1 : Scope
  Sum : Sum  Inputs=|++
  OP_setpoint_percent : Outport
  tag scope: Delta_P_percent=global, FR_reg_Starting_Setpoint_percent=global, Op_setpoint_percent=global, Over_Freq_En=global, Under_Freq_En=global
  wires:
  Constant5/1 -> Mux/3
  Mux/1 -> MATLAB Function5/1(u)
  Under_Freq_En/1 -> [Under_Freq_En], Mux/1
  U_Delta_P/1 -> Mux/2
  Mux1/1 -> MATLAB Function1/1(u)
  Over_Freq_En/1 -> [Over_Freq_En], Mux1/1, Mux5/1, Memory/1, Mux2/1
  O_Delta_P/1 -> Mux1/2
  MATLAB Function5/1(y) -> Mux1/3
  Mux2/1 -> MATLAB Function2/1(u)
  Memory/1 -> Mux2/2
  FB_measure_percent/1 -> Mux4/2, Mux3/2
  FR_reg_Starting_Setpoint_percent/1 -> Mux3/3
  MATLAB Function2/1(y) -> Mux3/1, Mux4/1
  Mux3/1 -> MATLAB Function3/1(u)
  MATLAB Function3/1(y) -> [FR_reg_Starting_Setpoint_percent]  "FR_reg_Starting_Setpoint_percent"
  MATLAB Function1/1(y) -> [Delta_P_percent]  "Delta_P_percent"
  Op_setpoint_percent/1 -> Mux4/3
  Mux4/1 -> MATLAB Function4/1(u)
  MATLAB Function4/1(y) -> [Op_setpoint_percent]  "Op_setpoint_Percent"
  CURTAILED_MODE_EN/1 -> Mux5/2
  Mux5/1 -> MATLAB Function6/1(u)
  [FR_reg_Starting_Setpoint_percent] -> Min/1
  Setpoint_percent/1 -> Min/2, Mux6/3
  Min/1 -> Mux6/2
  MATLAB Function6/1(y) -> Mux6/1
  Mux6/1 -> Scope1/1, MATLAB Function7/1(u)
  MATLAB Function7/1(y) -> Sum/1
  [Delta_P_percent] -> Sum/2
  Sum/1 -> OP_setpoint_percent/1, [Setpoint_percent]  "Setpoint_percent"
  Mux7/1 -> MATLAB Function8/1(u)
  [Under_Freq_En] -> Mux7/1
  [Over_Freq_En] -> Mux7/2
  Mux8/1 -> Scope/1, MATLAB Function9/1(u)
  MATLAB Function8/1(y) -> Mux8/1
  [Setpoint_percent] -> Mux8/2
  [Op_setpoint_percent] -> Mux8/3

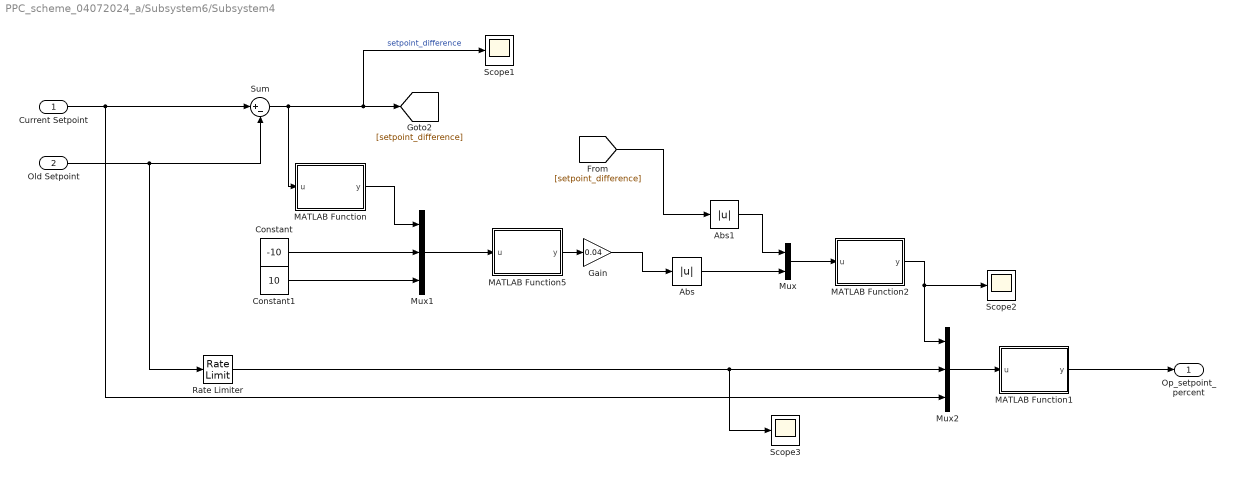
== system PPC_scheme_04072024_a/Subsystem6/Subsystem4 ==
  Current Setpoint : Inport
  Old Setpoint : Inport  Port=2
  Abs : Abs  SaturateOnIntegerOverflow=off
  Abs1 : Abs  SaturateOnIntegerOverflow=off
  Constant : Constant  Value=-10
  Constant1 : Constant  Value=10
  Gain : Gain  Gain=0.04
  MATLAB Function : MATLAB Function  TreatAsAtomicUnit=on
  MATLAB Function1 : MATLAB Function  TreatAsAtomicUnit=on
  MATLAB Function2 : MATLAB Function  TreatAsAtomicUnit=on
  MATLAB Function5 : MATLAB Function  TreatAsAtomicUnit=on
  Mux : Mux  Inputs=2
  Mux1 : Mux  Inputs=3
  Mux2 : Mux  Inputs=3
  Rate Limiter : RateLimiter  RisingSlewLimit=0.4  FallingSlewLimit=-0.4  SampleTimeMode=inherited
  Scope1 : Scope
  Scope2 : Scope
  Scope3 : Scope
  Sum : Sum  Inputs=|+-
  Op_setpoint_percent : Outport
  wires:
  Sum/1 -> MATLAB Function/1(u), Scope1/1, [setpoint_difference]  "setpoint_difference"
  Current Setpoint/1 -> Mux2/3, Sum/1
  Old Setpoint/1 -> Rate Limiter/1, Sum/2
  Constant/1 -> Mux1/2
  Constant1/1 -> Mux1/3
  MATLAB Function/1(y) -> Mux1/1
  Mux1/1 -> MATLAB Function5/1(u)
  Gain/1 -> Abs/1
  [setpoint_difference] -> Abs1/1
  Mux/1 -> MATLAB Function2/1(u)
  Rate Limiter/1 -> Scope3/1, Mux2/2
  Mux2/1 -> MATLAB Function1/1(u)
  MATLAB Function2/1(y) -> Scope2/1, Mux2/1
  MATLAB Function1/1(y) -> Op_setpoint_percent/1
  Abs1/1 -> Mux/1
  MATLAB Function5/1(y) -> Gain/1
  Abs/1 -> Mux/2

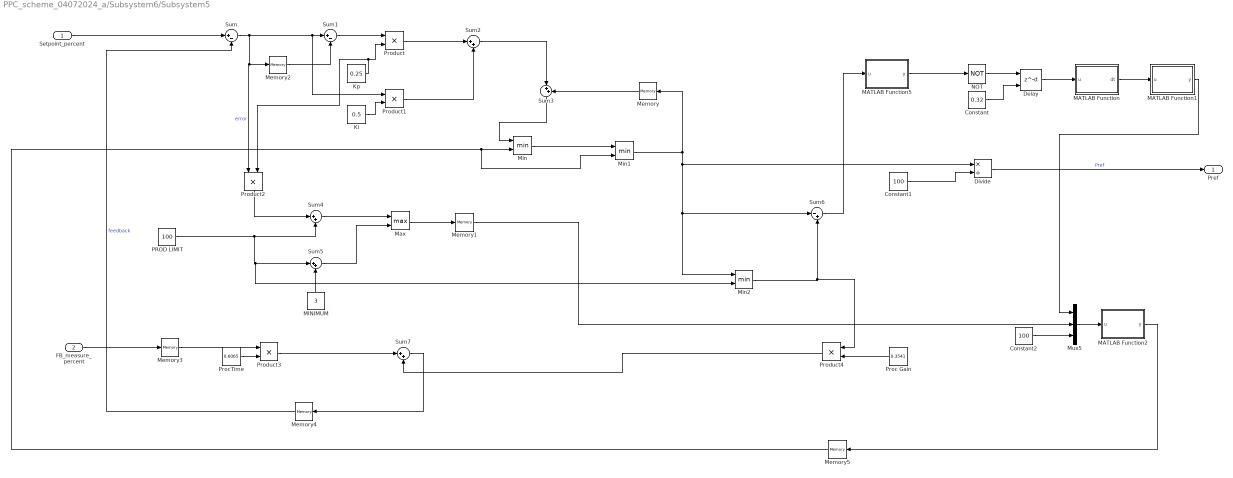
== system PPC_scheme_04072024_a/Subsystem6/Subsystem5 ==
  Setpoint_percent : Inport
  FB_measure_percent : Inport  Port=2
  Constant : Constant  Value=0.32
  Constant1 : Constant  Value=100
  Constant2 : Constant  Value=100
  Delay : Delay  DelayLengthSource=Input port  DelayLength=0.32  InitialCondition=1
      settings: InputPortMap=u0,p1
  Divide : Product  Inputs=*/
  Ki : Constant  Value=0.5
  Kp : Constant  Value=0.25
  MATLAB Function : MATLAB Function  TreatAsAtomicUnit=on
  MATLAB Function1 : MATLAB Function  TreatAsAtomicUnit=on
  MATLAB Function2 : MATLAB Function  TreatAsAtomicUnit=on
  MATLAB Function5 : MATLAB Function  TreatAsAtomicUnit=on
  MINIMUM : Constant  Value=3
  Max : MinMax  Function=max  Inputs=2
  Memory{,1..5} (6 alike) : Memory
  Min : MinMax  Inputs=2
  Min1 : MinMax  Inputs=2
  Min2 : MinMax  Inputs=2
  Mux5 : Mux  Inputs=3
  NOT : Logic  Operator=NOT  IconShape=distinctive  AllPortsSameDT=off  OutDataTypeStr=boolean
  PROD LIMIT : Constant  Value=100
  Proc Gain : Constant  Value=0.3541
  ProcTime : Constant  Value=0.6065
  Product{,1..4} (5 alike) : Product
  Sum : Sum  Inputs=|+-
  Sum1 : Sum  Inputs=|+-
  Sum{2..5,7} (5 alike) : Sum  Inputs=|++
  Sum6 : Sum  Inputs=|-+
  Pref : Outport
  wires:
  Sum/1 -> Product1/1, Sum1/1, Memory2/1, Product2/1  "error"
  Memory2/1 -> Sum1/2
  Setpoint_percent/1 -> Sum/1
  Sum1/1 -> Product/1
  Kp/1 -> Product/2, Product2/2
  Ki/1 -> Product1/2
  Product/1 -> Sum2/1
  Product1/1 -> Sum2/2
  Memory5/1 -> Min1/2, Min/2
  Sum2/1 -> Sum3/1
  Sum3/1 -> Min/1
  Min/1 -> Min1/1
  Memory/1 -> Sum3/2
  Min1/1 -> Sum6/1, Min2/1, Divide/1, Memory/1
  Product2/1 -> Sum4/1
  PROD LIMIT/1 -> Min2/2, Sum5/1, Sum4/2
  MINIMUM/1 -> Sum5/2
  Sum4/1 -> Max/1
  Sum5/1 -> Max/2
  Max/1 -> Memory1/1
  Min2/1 -> Product4/1, Sum6/2
  Sum6/1 -> MATLAB Function5/1(u)
  MATLAB Function5/1(y) -> NOT/1
  Delay/1 -> MATLAB Function/1(u)
  MATLAB Function/1(dt) -> MATLAB Function1/1(u)
  NOT/1 -> Delay/1
  Constant/1 -> Delay/2
  Constant1/1 -> Divide/2
  Divide/1 -> Pref/1  "Pref"
  FB_measure_percent/1 -> Memory3/1
  Memory3/1 -> Product3/1
  ProcTime/1 -> Product3/2
  Product3/1 -> Sum7/1
  Proc Gain/1 -> Product4/2
  Product4/1 -> Sum7/2
  Sum7/1 -> Memory4/1
  Memory4/1 -> Sum/2  "feedback"
  MATLAB Function1/1(y) -> Mux5/1
  Memory1/1 -> Mux5/2
  Constant2/1 -> Mux5/3
  Mux5/1 -> MATLAB Function2/1(u)
  MATLAB Function2/1(y) -> Memory5/1

== matlab function PPC_scheme_04072024_a/Subsystem6/Subsystem3/MATLAB Function3 ==
  data: u input; y output
function y = select(u)
if u(1)==1
    y=u(2);
else
    y=u(3);
end

== matlab function PPC_scheme_04072024_a/Subsystem6/Subsystem3/MATLAB Function4 ==
  data: u input; y output
function y = select(u)
if u(1)==1
    y=u(2);
else
    y=u(3);
end

== matlab function PPC_scheme_04072024_a/Subsystem6/Subsystem3/MATLAB Function6 ==
  data: u input; y output
function y = and(u)
if u(1)==1 && u(2)==1
    y=1;
else
    y=0;
end

== matlab function PPC_scheme_04072024_a/Subsystem6/Subsystem3/MATLAB Function7 ==
  data: u input; y output
function y = select(u)
if u(1)==1
    y=u(2);
else
    y=u(3);
end

== matlab function PPC_scheme_04072024_a/Subsystem6/Subsystem3/MATLAB Function8 ==
  data: u input; y output
function y = or(u)
if u(1)==1 || u(2)==1
    y=1;
else
    y=0;
end

== matlab function PPC_scheme_04072024_a/Subsystem6/Subsystem1/MATLAB Function ==
  data: u input; y output
function y = selectpos(u)
if u(1)>=u(2)
    y=1;
else
    y=0;
end

== matlab function PPC_scheme_04072024_a/Subsystem6/Subsystem3/MATLAB Function9 ==
  data: u input; y output
function y = select(u)
if u(1,1)==0
    y=u(2,1);
else
    y=u(3,1);
end

== matlab function PPC_scheme_04072024_a/Subsystem6/Subsystem4/MATLAB Function ==
  data: u input; y output
function y = negative(u)
if u<0
    y=1;
else
    y=0;
end

== matlab function PPC_scheme_04072024_a/Subsystem6/Subsystem4/MATLAB Function5 ==
  data: u input; y output
function y = select(u)
if u(1)==1
    y=u(2);
else
    y=u(3);
end

== matlab function PPC_scheme_04072024_a/Subsystem6/Subsystem4/MATLAB Function2 ==
  data: u input; y output
function y = selectpos(u)
if u(1)>=u(2)
    y=1;
else
    y=0;
end

== matlab function PPC_scheme_04072024_a/Subsystem6/Subsystem4/MATLAB Function1 ==
  data: u input; y output
function y = select(u)
if u(1)==1
    y=u(2);
else
    y=u(3);
end

== matlab function PPC_scheme_04072024_a/Subsystem6/Subsystem5/MATLAB Function5 ==
  data: u input; y output
function y = selectabs(u)
if abs(u)>0.1
    y=1;
else
    y=0;
end

== matlab function PPC_scheme_04072024_a/Subsystem6/Subsystem5/MATLAB Function ==
  data: u input; dt output
function dt = dtcomputation(u)
if u>0.5
    dt=1;
else
    dt=0;
end

== matlab function PPC_scheme_04072024_a/Subsystem6/Subsystem5/MATLAB Function1 ==
  data: u input; y output
function y = reset(u)

y = 1-u;

== matlab function PPC_scheme_04072024_a/Subsystem6/Subsystem5/MATLAB Function2 ==
  data: u input; y output
function y = select(u)
if u(1)==1
    y=u(2);
else
    y=u(3);
end

== matlab function PPC_scheme_04072024_a/Subsystem5/Subsystem3/MATLAB Function ==
  data: u input; y output
function y = multiselector(u)
if u(1)==1
    y=u(2);
elseif u(1)==2
    y=u(3);
else u(1)==3
    y=u(4);
end

== matlab function PPC_scheme_04072024_a/Subsystem6/Subsystem1/MATLAB Function2 ==
  data: u input; y output
function y = selectpos(u)
if u(1)>=u(2)
    y=1;
else
    y=0;
end

== matlab function PPC_scheme_04072024_a/Subsystem5/Subsystem4/MATLAB Function4 ==
  data: u input; y output
function y = select(u)
if u(1)==1
    y=u(2);
else
    y=u(3);
end

== matlab function PPC_scheme_04072024_a/Subsystem5/Subsystem4/MATLAB Function ==
  data: u input; y output
function y = update(u)
if u(1)>=u(2)
    y=1;
else
    y=0;
end

== matlab function PPC_scheme_04072024_a/Subsystem5/Subsystem4/MATLAB Function1 ==
  data: u input; y output
function y = select(u)
if u(1)==1
    y=u(2);
else
    y=u(3);
end

== matlab function PPC_scheme_04072024_a/Subsystem6/Subsystem1/MATLAB Function3 ==
  data: u input; y output
function y = and(u)
if u(1)==1 && u(2)==1
    y=1;
else
    y=0;
end

== matlab function PPC_scheme_04072024_a/Subsystem6/Subsystem1/MATLAB Function4 ==
  data: u input; y output
function y = select(u)
if u(1)==1
    y=u(2);
else
    y=u(3);
end

== matlab function PPC_scheme_04072024_a/Subsystem6/Subsystem2/MATLAB Function ==
  data: u input; y output
function y = selectneg(u)
if u(1)<=u(2)
    y=1;
else
    y=0;
end

== matlab function PPC_scheme_04072024_a/Subsystem6/Subsystem2/MATLAB Function3 ==
  data: u input; y output
function y = fcn(u)
if u(1)==0 && u(2)==1
    y=1;
else
    y=0;
end

== matlab function PPC_scheme_04072024_a/Subsystem6/Subsystem2/MATLAB Function1 ==
  data: u input; y output
function y = hold(u)
reset_time=0;
if u(2)==0 && u(3)==1
    reset_time=u(1);
else
    reset_time=-9999;
end
reset_delay=1;
if u(1)-reset_time< reset_delay
    y=u(1);
else
    if u(2)>0
        y=1;
    else
        y=0;
    end
end

== matlab function PPC_scheme_04072024_a/Subsystem6/Subsystem2/MATLAB Function2 ==
  data: u input; y output
function y = selectneg(u)
if u(1)<=u(2)
    y=1;
else
    y=0;
end

== matlab function PPC_scheme_04072024_a/Subsystem6/Subsystem1/MATLAB Function1 ==
  data: u input; y output
function y = hold(u)
reset_time=0;
if u(2)==0 && u(3)==1
    reset_time=u(1);
else
    reset_time=-9999;
end
reset_delay=1;
if u(1)-reset_time< reset_delay
    y=u(1);
else
    if u(2)>0
        y=1;
    else
        y=0;
    end
end

== matlab function PPC_scheme_04072024_a/Subsystem6/Subsystem2/MATLAB Function4 ==
  data: u input; y output
function y = fcn(u)
if u(1)==1 && u(2)==1
    y=1;
else
    y=0;
end

== matlab function PPC_scheme_04072024_a/Subsystem6/Subsystem2/MATLAB Function5 ==
  data: u input; y output
function y = select(u)
if u(1)==1
    y=u(2);
else
    y=u(3);
end

== matlab function PPC_scheme_04072024_a/Subsystem6/Subsystem3/MATLAB Function5 ==
  data: u input; y output
function y = select(u)
if u(1)==1
    y=u(2);
else
    y=u(3);
end

== matlab function PPC_scheme_04072024_a/Subsystem6/Subsystem3/MATLAB Function1 ==
  data: u input; y output
function y = select(u)
if u(1)==1
    y=u(2);
else
    y=u(3);
end

== matlab function PPC_scheme_04072024_a/Subsystem6/Subsystem3/MATLAB Function2 ==
  data: u input; y output
function y = select(u)
if u(1)==1 && u(2)==0
    y=1;
else
    y=0;
end
